simulink model "OSWEC"  (R2020a)
settings: Solver=ode4  StartTime=0  StopTime=200  FixedStep=0.01  MaxStep=0.01  RelTol=1e-3  EnableMultiTasking=on
values from neighbouring files (symbols this model uses):
  Bv = viscLDamp + ptoDamp + viscQDamp    [ptoSimInputFile.m]    (also in userDefinedFunctions.m)
  controller = struct()    [ptoSimInputFile.m]
  ptosim = ptoSimClass('Non-Compressible Fluid Hydraulic')    [ptoSimInputFile.m]
  R = body(1).hydroData.hydro_coeffs.radiation_damping.all(5,5,w_ind).*simu.rho*2*pi/waves.T    [ptoSimInputFile.m]    (also in userDefinedFunctions.m)
  simu = simulationClass()    [wecSimInputFile.m]
  waves = waveClass('irregular')    [wecSimInputFile.m]
undefined symbols (not defined in the file or in its folder): body, constraint, pto, X, Y, Z
libraries: nesl_utility x22, sm_lib x16, WECSim_Lib x10, PTOSim_Lib x3, vrlib x1, simulink x1
(part 4 of 4)

== matlab function OSWEC/Flap/Hydrodynamic Body/Morison Element and ViscousDampingForceCalculation/Morison Element Variant Subsystem/Morison Element On/Regular Wave Morison Force/MATLAB Function ==
  data: z input; f output; r input; Vel input; Accel input; Disp input; Area input; Cd input; Vol input; Ca input; Time input; rho input; waveDir input; waterDepth input; k input; w input; A input; rampTime input; g input; currentSpeed input; currentDirection input; currentDepth input; currentOption input; simuMorison input
function f = fcn(z,r,Vel,Accel,Disp,Area,Cd,Vol,Ca,Time,rho,waveDir,waterDepth,k,w,A,rampTime,g,currentSpeed,currentDirection,currentDepth,currentOption,simuMorison)
% This function calculates the Morison element force for the regular wave
% case.
[rr,~]=size(r);
FMt = zeros(rr,6);
for ii = 1:rr
    % Calculate Rotation Matrix
    RotMax      = [cos(Disp(5))*cos(Disp(6)) , cos(Disp(4))*sin(Disp(6)) + sin(Disp(4))*sin(Disp(5))*cos(Disp(6)) , sin(Disp(4))*sin(Disp(6)) - cos(Disp(4))*sin(Disp(5))*sin(Disp(6));...
                   -cos(Disp(5))*sin(Disp(6)), cos(Disp(4))*cos(Disp(6)) -  sin(Disp(4))*sin(Disp(5))*sin(Disp(6)), sin(Disp(4))*cos(Disp(6)) + cos(Disp(4))*sin(Disp(5))*sin(Disp(6));...
                   sin(Disp(5))              , -sin(Disp(4))*cos(Disp(5))                                         , cos(Disp(4))*cos(Disp(5))                                        ];
    % Rotate Cartesian
    rRot        = mtimes(RotMax,r(ii,:).')';
    Dispt       = [Disp(1),Disp(2),Disp(3)];
    ShiftCg     = Dispt + rRot;
    zRot        = mtimes(RotMax,z(ii,:)')';
    % Update translational and rotational velocity
    % w refers to \omega = rotational velocity
    Velt        = [Vel(4),Vel(5),Vel(6)];
    wxr         = cross(Velt,r(ii,:));
    %
    switch currentOption
        case 0
            currentSpeedDepth = currentSpeed;
        case 1
            if ShiftCg(3) > -currentDepth
                currentSpeedDepth = currentSpeed*(1 + ShiftCg(3)/currentDepth)^(1/7);
            else
                currentSpeedDepth = 0;
            end
        case 2
            if ShiftCg(3) > -currentDepth
                currentSpeedDepth = currentSpeed*(1 + ShiftCg(3)/currentDepth);
            else
                currentSpeedDepth = 0;
            end
        otherwise
            currentSpeedDepth = 0;
    end
    % Ramp Time
    if Time <= rampTime
        curramp     = currentSpeedDepth*(1 + cos(pi + pi/rampTime*Time))/2;
    else
        curramp     = currentSpeedDepth;
    end
    %Vel should be a column vector
    Vel2            = [Vel(1),Vel(2),Vel(3)] + wxr + [curramp*cosd(currentDirection),curramp*sind(currentDirection),0];
    % Update translational and rotational acceleration
    % dotw refers to \dot{\omega} = rotational acceleration
    Accelt          = [Accel(4),Accel(5),Accel(6)];
    dotwxr          = cross(Accelt,r(ii,:));
    wxwxr           = cross(Velt,wxr);
    Accel2          = [Accel(1),Accel(2),Accel(3)] + dotwxr + wxwxr;
    %% Calculate Orbital Velocity
    waveDirRad      = waveDir*pi/180;
    phaseArg        = w*Time - k*(ShiftCg(1)*cos(waveDirRad) + ShiftCg(2)*sin(waveDirRad));
    % Vertical Variation
    kh              = k*waterDepth;    
    kz              = k*ShiftCg(3);
    if kh > pi  % Deep water wave
        coeffHorz   = exp(kz);
        coeffVert   = coeffHorz;
    else        % Shallow & Intermediate Depth
        coeffHorz   = cosh(kz + kh)/cosh(kh);
        coeffVert   = sinh(kz + kh)/cosh(kh);
    end
    % Ramp Time
    if Time <= rampTime
        ramp        = (A/2)*(1 + cos( pi + pi/rampTime*Time));
    else
        ramp        = A;
    end
    % Orbital Velocity
    uV              =  ramp*coeffHorz*cos(phaseArg)*g*k*(1/w)*cos(waveDirRad);
    vV              =  ramp*coeffHorz*cos(phaseArg)*g*k*(1/w)*sin(waveDirRad);
    wV              = -ramp*coeffVert*sin(phaseArg)*g*k*(1/w);
    fluidV          = [uV, vV, wV];
    % Orbital Acceleration
    uA              = -ramp*coeffHorz*sin(phaseArg)*g*k*cos(waveDirRad);
    vA              = -ramp*coeffHorz*sin(phaseArg)*g*k*sin(waveDirRad);
    wA              = -ramp*coeffVert*cos(phaseArg)*g*k;
    fluidA          = [uA, vA, wA];
    if simuMorison == 2
        %% Decompose Fluid Velocity
        % Tangential Velocity
        vT          = ((dot(zRot,fluidV))/(norm(zRot)^2))*zRot;
        % Normal Velocity
        vN          = fluidV-vT;
        %% Decompose Fluid Acceleration
        AT          = ((dot(zRot,fluidA))/(norm(zRot)^2))*zRot;
        % Normal Acceleration
        AN          = fluidA-AT;
        %% Decompose Body Velocity
        % Tangential Velocity
        Vel2T       = ((dot(zRot,Vel2))/(norm(zRot)^2))*zRot;
        % Normal Velocity
        Vel2N       = Vel2-Vel2T;
        %% Decompose Body Acceleration
        Accel2T     = ((dot(zRot,Accel2))/(norm(zRot))^2)*zRot;
        % Normal Acceleration
        Accel2N     = Accel2-Accel2T;
        %% Morison Equation
        % Forces from velocity drag
        FdN         = (1/2)*rho*Cd(ii,1)*Area(ii,1)*(vN-Vel2N)*norm(vN-Vel2N);    
        FdT         = (1/2)*rho*Cd(ii,2)*Area(ii,2)*(vT-Vel2T)*norm(vT-Vel2T);
        Fd          = FdT + FdN;
        % Forces from body acceleration inertia on the Morison Element
        FiN         = rho*Vol(ii,:)*Ca(ii,1)*(AN - Accel2N);
        FiT         = rho*Vol(ii,:)*Ca(ii,2)*(AT - Accel2T);
        Fbi         = FiN + FiT;
        % Forces from fluid acceleration inertia on the Morison Element
        Ffi         = rho*Vol(ii,:)*(fluidA);
        % Summation of inertial forces on the Morison Element
        Fi          = Ffi + Fbi;
        % Total Force from the Morison Element
        F           = Fi + Fd;
    else
        %% Added inertia and drag forces
        areaRot     = abs(mtimes(Area(ii,:),RotMax));
        CdRot       = mtimes(abs(Cd(ii,:)),RotMax);
        CaRot       = abs(mtimes(Ca(ii,:),RotMax));
        % Forces from velocity drag
        uVdiff      = uV - Vel2(1); FxuV = (1/2)*abs(uVdiff)*uVdiff*rho*CdRot(1)*areaRot(1);
        vVdiff      = vV - Vel2(2); FxvV = (1/2)*abs(vVdiff)*vVdiff*rho*CdRot(2)*areaRot(2);
        wVdiff      = wV - Vel2(3); FxwV = (1/2)*abs(wVdiff)*wVdiff*rho*CdRot(3)*areaRot(3);
        % Forces from body acceleration inertia
        uAdiff      = uA - Accel2(1); FxuA = uAdiff*rho*Vol(ii,:)*CaRot(1);
        vAdiff      = vA - Accel2(2); FxvA = vAdiff*rho*Vol(ii,:)*CaRot(2);
        wAdiff      = wA - Accel2(3); FxwA = wAdiff*rho*Vol(ii,:)*CaRot(3);
        % Forces from fluid acceleration inertia
        FxuAf       = uA*Vol(ii,:)*rho;
        FxvAf       = vA*Vol(ii,:)*rho;
        FxwAf       = wA*Vol(ii,:)*rho;
        % Total Force from the Morison Element
        F           = [FxuV + FxuA + FxuAf,...
                       FxvV + FxvA + FxvAf,...
                       FxwV + FxwA + FxwAf];
    end
    % Determine if the Morison Element point of application goes above the
    % mean water line and does not consider the local surface elevation.
    if ShiftCg(3) > 0
        F           = [0, 0, 0];
        M           = [0, 0, 0];
        FMt(ii,:)   = [F,M];
    else
        % Calculate the moment about the center of gravity for each Morison Element
        M           = cross(rRot,F);
        FMt(ii,:)   = [F,M];
    end
end
f      = 0.*Vel;
f(1:6) = [sum(FMt(:,1));sum(FMt(:,2));sum(FMt(:,3));sum(FMt(:,4));sum(FMt(:,5));sum(FMt(:,6))];
end

== matlab function OSWEC/Flap/Hydrodynamic Body/Hydrostatic Restoring Force Calculation/Linear and Nonlinear Restoring Force Variant Subsystem/Nonlinear Hydrostatic Restoring Force/Restoring Forces ==
  data: x input; elv input; center input; f output; tnorm input; area input; rho input; g input; cg input; p output; mass input
function [f,p]  = nonLinearBuoyancy(x,elv,center,tnorm,area,rho,g,cg,mass)
% Function to calculate buoyancy force and moment on a triangulated surface
% NOTE: This function assumes that the STL file is imported with its CG at 0,0,0
[f,p] = calc_buoyancy(x,elv,center,tnorm,area,rho,g,cg);
f = -f + [0 0 g*mass 0 0 0]';
end


function [f,p] = calc_buoyancy(x,elv,center,tnorm,area,rho,g,cg)
% Function to apply translation and rotation and calculate forces

% Compute new tri coords after cog rotation and translation
center = rotateXYZ(center,[1 0 0],x(4));
center = rotateXYZ(center,[0 1 0],x(5));
center = rotateXYZ(center,[0 0 1],x(6));
center = offsetXYZ(center,x);
center = offsetXYZ(center,cg);
% Compute new normal vectors coords after cog rotation
tnorm = rotateXYZ(tnorm,[1 0 0],x(4));
tnorm = rotateXYZ(tnorm,[0 1 0],x(5));
tnorm = rotateXYZ(tnorm,[0 0 1],x(6));

% Calculate the hydrostatic forces
av = tnorm .* [area area area];
[f,p]=fHydrostatic(center,elv,x(1:3)+cg,av,rho,g);
end

function [f,p] = fHydrostatic(center,elv,instcg,av,rho,g)
% Function to calculate the force and moment about the cog due to hydrostatic pressure
f = zeros(6,1);

% Zeor out regions above the mean free surface
z=center(:,3); z((z-elv)>0)=0;

% Calculate the hydrostatic pressure at each triangle center
pressureVect = rho*g.*[-z -z -z].*-av;
p = rho*g.*-z;
% Compute force about cog
f(1:3) = sum(pressureVect);

tmp1 = ones(length(center(:,1)),1);
tmp2 = tmp1*instcg';
center2cgVec = center-tmp2;

f(4:6)= sum(cross(center2cgVec,pressureVect));
end

== matlab function OSWEC/Flap/Hydrodynamic Body/Wave Diffraction and Excitation Force Calculation/Linear Wave Excitation Force Variant Subsystem/Irregular Wave NonLinearYaw/MATLAB Function ==
  data: A input; w input; dofGRD input; dirGRD input; wGRD input; fEHRE input; fEHIM input; Fext output; fEHMD input; phaseRand input; dw input; time input; WaveDir input; WaveSpread input; Disp input; intThresh input; prevYaw input; relYawLast output; prevCoeffMD input; prevCoeffRE input; prevCoeffIM input; coeffsLastMD output; coeffsLastRE output; coeffsLastIM output
function [Fext,relYawLast,coeffsLastMD,coeffsLastRE,coeffsLastIM] = fcn(A,w,dofGRD,dirGRD,wGRD,fEHRE,fEHIM, fEHMD, phaseRand,dw,time,WaveDir,WaveSpread, Disp, intThresh, prevYaw, prevCoeffMD, prevCoeffRE, prevCoeffIM)
%#codegen
% Fext is the excitation force output, relYawLast is the angle of relative
% yaw at which that last interpolation was performed. If the current
% relative yaw angle - last interpolated > threshold, the interpolation is
% performed again. To interpolate every time step, let threshold=0.

% caseFlag is for debug, delete when satisfied
A1=bsxfun(@plus,w*time,pi/2);
%initialize outputs
Fext = zeros(1,6);
relYawLast=0;
coeffsLastMD=zeros(length(w),6);
coeffsLastRE=zeros(length(w),6);
coeffsLastIM=zeros(length(w),6);

for ii=1:length(WaveDir)
    relYaw=WaveDir(ii)-(Disp(6)*180/pi); % relative yaw angle
    phaseRandint=phaseRand(:,ii);
    WaveSpreadint=WaveSpread(ii);
    
       % compare relYaw to available WaveDir data
        if relYaw>max(dirGRD(1,:,1)) % handle interpolation out of BEM range by wrapping other bound
            [~,idx]=min(dirGRD(1,:,1),[],2); % 
            dirGRD(:,idx,:)=dirGRD(:,idx,:)+360;
            [dirGRD,I]=sort(dirGRD,2); % grid must be in ascending order
                      
        elseif relYaw<min(dirGRD(1,:,1))
            [~,idx]=max(dirGRD(1,:,1),[],2); % 
            dirGRD(:,idx,:)=dirGRD(:,idx,:)-360;  
            [dirGRD,I]=sort(dirGRD,2); % grid must be in ascending order

        else 
            I=1:length(dirGRD(1,:,1));
        end
    
    if abs(relYaw-prevYaw)>intThresh && min(abs(relYaw-dirGRD(1,:,1)))>intThresh% interpolate for nonlinear yaw 
            
        % performs 1D interpolation in wave direction
        fExtMDint=interpn(dofGRD,dirGRD,wGRD,fEHMD(:,I(1,:,1),:),dofGRD,relYaw*ones(size(dirGRD)),wGRD);
        fExtREint=interpn(dofGRD,dirGRD,wGRD,fEHRE(:,I(1,:,1),:),dofGRD,relYaw*ones(size(dirGRD)),wGRD);
        fExtIMint=interpn(dofGRD,dirGRD,wGRD,fEHIM(:,I(1,:,1),:),dofGRD,relYaw*ones(size(dirGRD)),wGRD);
        
        % permute for dimensional consistency with linear yaw
        fExtMDint=squeeze(permute(fExtMDint(:,1,:),[2 3 1]));
        fExtREint=squeeze(permute(fExtREint(:,1,:),[2 3 1]));
        fExtIMint=squeeze(permute(fExtIMint(:,1,:),[2 3 1]));
        
        relYawLast=relYaw;
        coeffsLastMD=fExtMDint;
        coeffsLastRE=fExtREint;
        coeffsLastIM=fExtIMint;
        
    elseif min(abs(relYaw-dirGRD(1,:,1)))>intThresh % significant yaw is present, but close to previous value
        fExtMDint=prevCoeffMD;
        fExtREint=prevCoeffRE;
        fExtIMint=prevCoeffIM;
        
        relYawLast=prevYaw;
        coeffsLastMD=prevCoeffMD;
        coeffsLastRE=prevCoeffRE;
        coeffsLastIM=prevCoeffIM;
        
    else    % significant yaw may be is present, but nearby BEM calculated data
        [~,idx]=min(abs(relYaw-dirGRD(1,:,1)));
        fExtMDint=squeeze(fEHMD(:,I(1,idx,1),:)).'; % maintains dimensional consistency
        fExtREint=squeeze(fEHRE(:,I(1,idx,1),:)).';
        fExtIMint=squeeze(fEHIM(:,I(1,idx,1),:)).';
        
        relYawLast=dirGRD(1,idx,1); % indices of dirGRD have already been resorted
        coeffsLastMD=fExtMDint;
        coeffsLastRE=fExtREint;
        coeffsLastIM=fExtIMint;
    end
    B1= sin(bsxfun(@plus,A1,phaseRandint));
    B11 = sin(bsxfun(@plus,w*time,phaseRandint));
    C0 = bsxfun(@times,A*WaveSpreadint,dw);
    C1 = sqrt(bsxfun(@times,A*WaveSpreadint,dw));
    D0 =bsxfun(@times,fExtMDint,C0);
    D1 =bsxfun(@times,fExtREint,C1);
    D11 = bsxfun(@times,fExtIMint,C1);
    E1 = D0+ bsxfun(@times,B1,D1);
    E11 = bsxfun(@times,B11,D11);
    Fext = Fext + sum(bsxfun(@minus,E1,E11));
end

== matlab function OSWEC/Flap/Hydrodynamic Body/Morison Element and ViscousDampingForceCalculation/Morison Element Variant Subsystem/Morison Element On/No Wave Morison Force/MorisonElement(s) ==
  data: z input; f output; r input; Vel input; Accel input; Disp input; Area input; Cd input; Vol input; Ca input; Time input; rho input; rampTime input; currentSpeed input; currentDirection input; currentDepth input; currentOption input; simuMorison input
function f = fcn(z,r,Vel,Accel,Disp,Area,Cd,Vol,Ca,Time,rho,rampTime,currentSpeed,currentDirection,currentDepth,currentOption,simuMorison)
% This function calculates the Morison element force for the no wave case.
[rr,~]=size(r);
FMt = zeros(rr,6);
for ii = 1:rr
    % Calculate Rotation Matrix
    RotMax = [cos(Disp(5))*cos(Disp(6)) , cos(Disp(4))*sin(Disp(6)) + sin(Disp(4))*sin(Disp(5))*cos(Disp(6)) , sin(Disp(4))*sin(Disp(6)) - cos(Disp(4))*sin(Disp(5))*sin(Disp(6));...
              -cos(Disp(5))*sin(Disp(6)), cos(Disp(4))*cos(Disp(6)) -  sin(Disp(4))*sin(Disp(5))*sin(Disp(6)), sin(Disp(4))*cos(Disp(6)) + cos(Disp(4))*sin(Disp(5))*sin(Disp(6));...
              sin(Disp(5))              , -sin(Disp(4))*cos(Disp(5))                                         , cos(Disp(4))*cos(Disp(5))                                        ];
    % Rotate Cartesian
    rRot    = mtimes(RotMax,r(ii,:).')';
    Dispt   = [Disp(1),Disp(2),Disp(3)];
    ShiftCg = Dispt + rRot;
    zRot    = mtimes(RotMax,z(ii,:)')';
    % Update translational and rotational velocity
    % w refers to \omega = rotational velocity
    Velt    = [Vel(4),Vel(5),Vel(6)];
    wxr     = cross(Velt,r(ii,:));
    %
    switch currentOption
        case 0
            currentSpeedDepth = currentSpeed;
        case 1
            if ShiftCg(3) > -currentDepth
                currentSpeedDepth = currentSpeed*(1 + ShiftCg(3)/currentDepth)^(1/7);
            else
                currentSpeedDepth = 0;
            end
        case 2
            if ShiftCg(3) > -currentDepth
                currentSpeedDepth = currentSpeed*(1 + ShiftCg(3)/currentDepth);
            else
                currentSpeedDepth = 0;
            end
        otherwise
            currentSpeedDepth = 0;
    end
    % Ramp Time
    if Time <= rampTime
        curramp        = currentSpeedDepth*(1 + cos(pi + pi/rampTime*Time))/2;
    else
        curramp        = currentSpeedDepth;
    end
    %Vel should be a column vector
    Vel2    = [Vel(1),Vel(2),Vel(3)] + wxr + [curramp*cosd(currentDirection),curramp*sind(currentDirection),0];
    % Update translational and rotational acceleration
    % dotw refers to \dot{\omega} = rotational acceleration
    Accelt  = [Accel(4),Accel(5),Accel(6)];
    dotwxr  = cross(Accelt,r(ii,:));
    wxwxr   = cross(Velt,wxr);
    Accel2  = [Accel(1),Accel(2),Accel(3)] + dotwxr + wxwxr;
    if simuMorison == 2
        %% Decompose Body Velocity
        % Tangential Velocity
        Vel2T           = ((dot(zRot,Vel2))/(norm(zRot))^2)*zRot;
        % Normal Velocity
        Vel2N           = Vel2-Vel2T;
        %% Decompose Body Acceleration
        Accel2T         = ((dot(zRot,Accel2))/(norm(zRot)^2))*zRot;
        % Normal Acceleration
        Accel2N         = Accel2-Accel2T;
        %% Morison Equation
        % Forces from velocity drag
        FdN             = (1/2)*rho*Cd(ii,1)*Area(ii,1)*norm(Vel2N)*(-Vel2N);
        FdT             = (1/2)*rho*Cd(ii,2)*Area(ii,2)*norm(Vel2T)*(-Vel2T);
        Fd              = FdT + FdN;
        % Forces from body acceleration inertia
        FiN             = rho*Vol(ii,:)*Ca(ii,1)*(-Accel2N);
        FiT             = rho*Vol(ii,:)*Ca(ii,2)*(-Accel2T);
        Fbi             = FiN + FiT;
        F               = Fbi + Fd;
    else
        %% Added inertia and drag forces
        areaRot     = abs(mtimes(Area(ii,:),RotMax));
        CdRot       = mtimes(abs(Cd(ii,:)),RotMax);
        CaRot       = abs(mtimes(Ca(ii,:),RotMax));
        % Forces from body velocity drag
        FxuV        = (1/2)*abs(-1*Vel2(1))*-1*Vel2(1)*rho*CdRot(1)*areaRot(1);
        FxvV        = (1/2)*abs(-1*Vel2(2))*-1*Vel2(2)*rho*CdRot(2)*areaRot(2);
        FxwV        = (1/2)*abs(-1*Vel2(3))*-1*Vel2(3)*rho*CdRot(3)*areaRot(3);
        % Forces from body acceleration inertia
        FxuA        = rho*Vol(ii,:)*CaRot(1)*-1*Accel2(1);
        FxvA        = rho*Vol(ii,:)*CaRot(2)*-1*Accel2(2);
        FxwA        = rho*Vol(ii,:)*CaRot(3)*-1*Accel2(3);
        % Sum the force contributions
        F           = [FxuV + FxuA,FxvV + FxvA,FxwV + FxwA];
    end
    % Determine if the Morison Element point of application goes above the
    % mean water line and does not consider the local surface elevation.
    if ShiftCg(3) > 0
        F           = [0, 0, 0];
        M           = [0, 0, 0];
        % Calculate the moment about the center of gravity for each Morison Element
        FMt(ii,:)   = [F,M];
    else
        % Calculate the moment about the center of gravity for each Morison Element
        M           = cross(rRot,F);
        FMt(ii,:)   = [F,M];
    end
end
f      = 0.*Vel;
f(1:6) = [sum(FMt(:,1));sum(FMt(:,2));sum(FMt(:,3));sum(FMt(:,4));sum(FMt(:,5));sum(FMt(:,6))];
end
